simulink model "main2"  (R2015a)
settings: Solver=ode3  StartTime=0.0  StopTime=inf  RelTol=1e-3
undefined symbols (not defined in the file): Rec, SDTV
libraries: embdlinuxlib x4, visionconversions x2, visionstatistics x1, visiontextngfix x1, visionanalysis x1
settings Model: SimulationMode=external  ExtModeTrigDuration=100  Creator=User  LastModifiedBy=User
settings OptimizationCC: OptimizeModelRefInitCode=on  LifeSpan=1
settings DebuggingCC: UnderspecifiedInitializationDetection=Classic  MergeDetectMultiDrivingBlocksExec=none
settings HardwareCC: ProdLargestAtomicInteger=Long  ProdLargestAtomicFloat=Double  ProdEndianess=LittleEndian  ProdHWDeviceType=ARM Compatible->ARM Cortex
settings RTWCC: SystemTargetFile=realtime.tlc  GenerateMakefile=off  TemplateMakefile=realtime.tmf  Description=Run on Target Hardware  RTWVerbose=off
settings ERTTargetCC: CombineOutputUpdateFcns=off  ExtModeMexArgs='192.168.15.103' 0 17725  ERTSrcFileBannerTemplate=realtime_code_template.cgt  ERTHdrFileBannerTemplate=realtime_code_template.cgt  ERTDataSrcFileTemplate=realtime_code_template.cgt  ERTDataHdrFileTemplate=realtime_code_template.cgt  ERTCustomFileTemplate=realtime_file_process.tlc

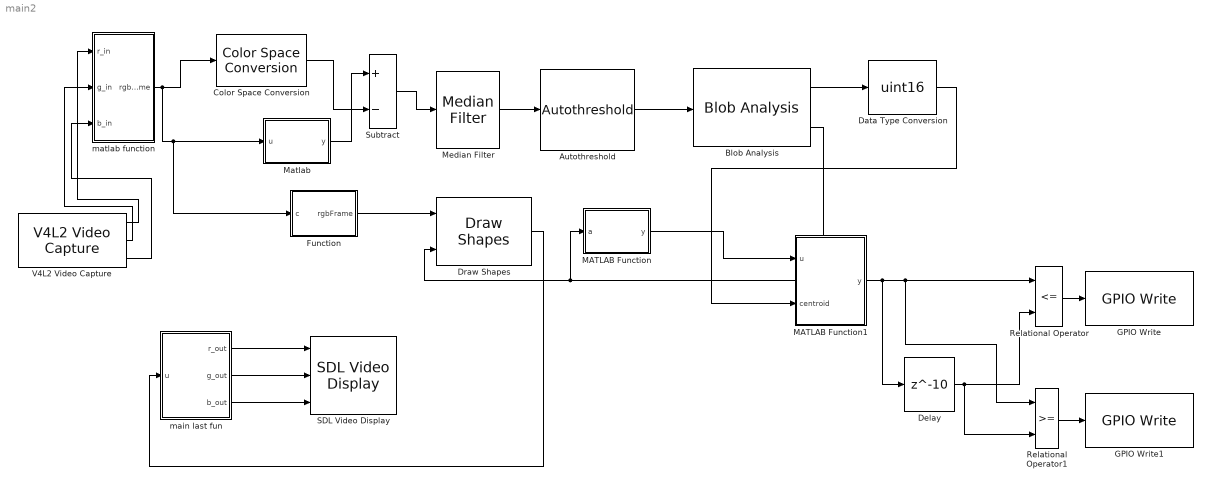
== system main2 ==
  " Function" : MATLAB Function  TreatAsAtomicUnit=on
  Autothreshold : visionconversions/Autothreshold  operator=>  threshOut=off  effMetricOut=off  userDefinedRange=off  umin=0  umax=255  outOfRngOpt=Warn and saturate  scaleThreshold=on  scaleFactor=1.15  P1Mode=Specify word length  P1WordLength=32  P1FracLength=30  P2Mode=Specify word length  P2WordLength=32  P2FracLength=22  P3Mode=Specify word length  P3WordLength=32  P3FracLength=14  P4Mode=Binary point scaling  P4WordLength=32  P4FracLength=15  Q1Mode=Specify word length  Q1WordLength=32  Q1FracLength=16  EMMode=Specify word length  EMWordLength=16  EMFracLength=14  roundingMode=Floor  overflowMode=off
  Blob Analysis : visionstatistics/Blob Analysis  Tag=vipblks_row_conv  area=off  centroid=on  bBox=on  majorAxis=off  minorAxis=off  angle=off  eccentricity=off  equivDiameterSq=off  extent=off  perimeter=off  maxBlobs=1  warnIfNumBlobsExceeded=on  isCount=off  useMinArea=on  minArea=600  useMaxArea=on  maxArea=3000  excludeBorderBlob=off  outDT=double  isOutVarDim=off  isFill=on  fillValues=-1  conn=8  isLabel=off  outputMode=Binary point scaling  outputWordLength=32  outputFracLength=16  firstCoeffMode=Binary point scaling  firstCoeffWordLength=16  firstCoeffFracLength=14  secondCoeffMode=Binary point scaling  secondCoeffWordLength=32  secondCoeffFracLength=16  accumMode=Binary point scaling  accumWordLength=32  accumFracLength=0  prodOutputMode=Binary point scaling  prodOutputWordLength=32  prodOutputFracLength=16  roundingMode=Floor  overflowMode=off
  Color Space Conversion : visionconversions/Color Space  Conversion  conversion=Obsolete  conversionActive=R'G'B' to intensity  wp_str=D65  rec=Rec. 601 (SDTV)  sys=1125/60/2:1  imagePorts=One multidimensional signal
  Data Type Conversion : DataTypeConversion  OutDataTypeStr=uint16
  Delay : Delay  DelayLength=10  InitialCondition=300
  Draw Shapes : visiontextngfix/Draw Shapes  shape=Rectangles  fill=on  lineWidth=1  fillClrSource=Specify via dialog  display=User-specified value  intensity=200  color=[255 0 0]  opacity=0.4  viewport=Entire image  antialiasing=off  inType=Obsolete  imagePorts=One multidimensional signal  prodOutputMode=Binary point scaling  prodOutputWordLength=32  prodOutputFracLength=14  memoryMode=Specify word length  memoryWordLength=16  memoryFracLength=14  roundingMode=Floor  overflowMode=off
  GPIO Write : embdlinuxlib/GPIO Write  board=Model B+  gpio=17  direction=Output  blockPlatform=Raspberry Pi
  GPIO Write1 : embdlinuxlib/GPIO Write  board=Model B+  gpio=27  direction=Output  blockPlatform=Raspberry Pi
  MATLAB Function : MATLAB Function  TreatAsAtomicUnit=on
  MATLAB Function1 : MATLAB Function  TreatAsAtomicUnit=on
  Matlab : MATLAB Function  TreatAsAtomicUnit=on
  Median Filter : visionanalysis/Median Filter  nghbood=[3 3]  outSize=Same as input port I  padType=Constant  padSrc=Specify via dialog  padVal=0  roundingMode=Floor  overflowMode=off
  Relational Operator : RelationalOperator  Operator=<=  OutDataTypeStr=boolean
  Relational Operator1 : RelationalOperator  OutDataTypeStr=boolean
  SDL Video Display : embdlinuxlib/SDL Video Display  pixelFormat=RGB  pixelOrder=Planar  rowMajor=on  blockPlatform=Raspberry Pi
  Subtract : Sum  Inputs=+-  SaturateOnIntegerOverflow=on  OutDataTypeStr=Inherit: Same as first input
  V4L2 Video Capture : embdlinuxlib/V4L2 Video Capture  m_devName='/dev/video0'  roi=[0, 0, 640, 480]  imSizeSelection=640x480  imSize=[640, 480]  pixelFormat=RGB  pixelOrder=Planar  sampleTime=1/10  simOutput=Colorbars  blockPlatform=Raspberry Pi
  main last fun : MATLAB Function  TreatAsAtomicUnit=on
  "matlab function " : MATLAB Function  TreatAsAtomicUnit=on
  wires:
  Blob Analysis/1 -> Data Type Conversion/1
  " Function"/1(rgbFrame) -> Draw Shapes/1
  Blob Analysis/2 -> MATLAB Function/1(a), Draw Shapes/2
  Subtract/1 -> Median Filter/1
  Median Filter/1 -> Autothreshold/1
  Autothreshold/1 -> Blob Analysis/1
  V4L2 Video Capture/1 -> "matlab function "/1(r_in)
  V4L2 Video Capture/2 -> "matlab function "/2(g_in)
  V4L2 Video Capture/3 -> "matlab function "/3(b_in)
  main last fun/1(r_out) -> SDL Video Display/1
  main last fun/3(b_out) -> SDL Video Display/3
  Color Space Conversion/1 -> Subtract/2
  Matlab/1(y) -> Subtract/1
  main last fun/2(g_out) -> SDL Video Display/2
  "matlab function "/1(rgb_Frame) -> " Function"/1(c), Matlab/1(u), Color Space Conversion/1
  Draw Shapes/1 -> main last fun/1(u)
  Relational Operator/1 -> GPIO Write/1
  Relational Operator1/1 -> GPIO Write1/1
  MATLAB Function/1(y) -> MATLAB Function1/1(u)
  Data Type Conversion/1 -> MATLAB Function1/2(centroid)
  MATLAB Function1/1(y) -> Delay/1, Relational Operator1/1, Relational Operator/1
  Delay/1 -> Relational Operator1/2, Relational Operator/2

== matlab function main2/main last fun ==
  data: u input; r_out output; g_out output; b_out output
function [r_out,g_out,b_out] = fcn(u)

r_out = u(:, :, 1);
g_out = u (:, :, 2);
b_out = u (:, :, 3);

== matlab function main2/matlab function  ==
  data: r_in input; rgb_Frame output; g_in input; b_in input
function rgb_Frame   = Threshaxis(r_in,g_in,b_in)
rgb_Frame= cat(3,r_in,g_in,b_in);
%rgb_Frame = flipdim(y,2);

== matlab function main2/ Function ==
  data: c input; rgbFrame output
function rgbFrame = fcn(c)
c(1:20,1:165,:) = 0;
rgbFrame=c;

== matlab function main2/Matlab ==
  data: u input; y output
function y = fcn(u)
%#codegen
y = u(:,:,1);

== matlab function main2/MATLAB Function1 ==
  data: u input; y output; centroid input
function y = fcn(u,centroid)
%#codegen

CentX =centroid(u,1);
y = CentX ;

== matlab function main2/MATLAB Function ==
  data: a input; y output
function y = fcn(a)
y = length(a(1,1));
